simulink model "model02_ol"  (Simulink 7.9)
settings: Solver=ode45  StartTime=0.0  StopTime=10.0  RelTol=1e-3
values from neighbouring files (symbols this model uses):
  T = 1/125    (= 0.008)    [M2_ol.m]
settings Model: Creator=ex16  LastModifiedBy=ex16

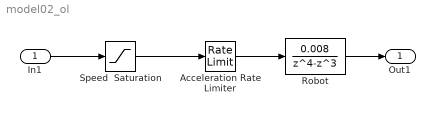
== system model02_ol ==
  In1 : Inport
  Acceleration Rate Limiter : RateLimiter  RisingSlewLimit=15  FallingSlewLimit=-15  SampleTimeMode=inherited
  Robot : DiscreteTransferFcn  Numerator=[0.008]  Denominator=[1 -1 0 0 0]  SampleTime=T
  Speed  Saturation : Saturate  UpperLimit=3.2  LowerLimit=-3.2  SampleTime=T
  Out1 : Outport
  wires:
  Robot/1 -> Out1/1
  Speed  Saturation/1 -> Acceleration Rate Limiter/1
  Acceleration Rate Limiter/1 -> Robot/1
  In1/1 -> Speed  Saturation/1
